simulink model "MODEL_TEMPLATE_NonLinear_Tire"  (Simulink 7.5)
settings: Solver=ode45  StartTime=0.0  StopTime=500  MaxStep=0.01  RelTol=1e-3
values from neighbouring files (symbols this model uses):
  U = NaN(2,nsteps)    [runscript.m]
undefined symbols (not defined in the file or in its folder): a, A, b, B, Caf, Car, Iz, m, steer_amplitude, tire_model_type
libraries: simulink x1
settings Model: Creator=snb10  LastModifiedBy=Matt
settings DataIOCC: SignalLoggingName=sigsOut
settings OptimizationCC: InlineInvariantSignals=on  InitFltsAndDblsToZero=on
settings DebuggingCC: SaveWithParameterizedLinksMsg=none  SignalResolutionControl=TryResolveAllWithWarning  SolverPrmCheckMsg=none  MultiTaskDSMMsg=warning  MultiTaskCondExecSysMsg=none  StrictBusMsg=None
settings HardwareCC: TargetUnknown=on
settings RTWCC: IncludeERTFirstTime=on
settings GRTTargetCC: TargetFcnLib=ansi_tfl_tmw.mat

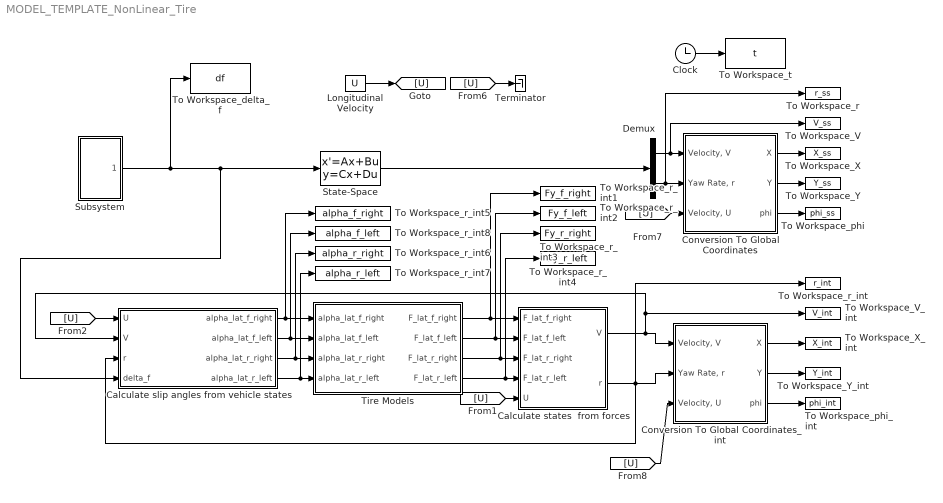
== system MODEL_TEMPLATE_NonLinear_Tire ==
  Calculate slip angles from vehicle states : Subsystem
  Calculate states  from forces : Subsystem
  Clock : Clock
      settings: Decimation=10
  Conversion To Global Coordinates : Subsystem
  Conversion To Global Coordinates_int : Subsystem
  Demux : Demux  Outputs=2
  Longitudinal Velocity : Constant  Value=U  OutDataType=sfix(16)  OutScaling=2^0
  State-Space : StateSpace  A=A  B=B(:,1)  C=eye(2)  D=zeros(2,1)
  Subsystem : Subsystem
  Terminator : Terminator
  Tire Models : Subsystem
  To Workspace_V : ToWorkspace  VariableName=V_ss  SampleTime=-1  SaveFormat=Array
  To Workspace_V_int : ToWorkspace  VariableName=V_int  SampleTime=-1  SaveFormat=Array
  To Workspace_X : ToWorkspace  VariableName=X_ss  SampleTime=-1  SaveFormat=Array
  To Workspace_X_int : ToWorkspace  VariableName=X_int  SampleTime=-1  SaveFormat=Array
  To Workspace_Y : ToWorkspace  VariableName=Y_ss  SampleTime=-1  SaveFormat=Array
  To Workspace_Y_int : ToWorkspace  VariableName=Y_int  SampleTime=-1  SaveFormat=Array
  To Workspace_delta_f : ToWorkspace  VariableName=df  SampleTime=-1  SaveFormat=Array
  To Workspace_phi : ToWorkspace  VariableName=phi_ss  SampleTime=-1  SaveFormat=Array
  To Workspace_phi_int : ToWorkspace  VariableName=phi_int  SampleTime=-1  SaveFormat=Array
  To Workspace_r : ToWorkspace  VariableName=r_ss  SampleTime=-1  SaveFormat=Array
  To Workspace_r_int : ToWorkspace  VariableName=r_int  SampleTime=-1  SaveFormat=Array
  To Workspace_r_int1 : ToWorkspace  VariableName=Fy_f_right  SampleTime=-1  SaveFormat=Array
  To Workspace_r_int2 : ToWorkspace  VariableName=Fy_f_left  SampleTime=-1  SaveFormat=Array
  To Workspace_r_int3 : ToWorkspace  VariableName=Fy_r_right  SampleTime=-1  SaveFormat=Array
  To Workspace_r_int4 : ToWorkspace  VariableName=Fy_r_left  SampleTime=-1  SaveFormat=Array
  To Workspace_r_int5 : ToWorkspace  VariableName=alpha_f_right  SampleTime=-1  SaveFormat=Array
  To Workspace_r_int6 : ToWorkspace  VariableName=alpha_r_right  SampleTime=-1  SaveFormat=Array
  To Workspace_r_int7 : ToWorkspace  VariableName=alpha_r_left  SampleTime=-1  SaveFormat=Array
  To Workspace_r_int8 : ToWorkspace  VariableName=alpha_f_left  SampleTime=-1  SaveFormat=Array
  To Workspace_t : ToWorkspace  VariableName=t  SampleTime=-1  SaveFormat=Array
  wires:
  Demux/1 -> Conversion To Global Coordinates/1("Velocity, V"), To Workspace_V/1
  Conversion To Global Coordinates/1(X) -> To Workspace_X/1
  Conversion To Global Coordinates/2(Y) -> To Workspace_Y/1
  Demux/2 -> Conversion To Global Coordinates/2("Yaw Rate, r"), To Workspace_r/1
  State-Space/1 -> Demux/1
  [U] -> Conversion To Global Coordinates/3("Velocity, U")
  Conversion To Global Coordinates/3(phi) -> To Workspace_phi/1
  Subsystem/1(delta_f) -> To Workspace_delta_f/1, State-Space/1, Calculate slip angles from vehicle states/4(delta_f)
  Clock/1 -> To Workspace_t/1
  Calculate states  from forces/1(V) -> Conversion To Global Coordinates_int/1("Velocity, V"), To Workspace_V_int/1, Calculate slip angles from vehicle states/2(V)
  Conversion To Global Coordinates_int/1(X) -> To Workspace_X_int/1
  Conversion To Global Coordinates_int/2(Y) -> To Workspace_Y_int/1
  [U] -> Conversion To Global Coordinates_int/3("Velocity, U")
  Conversion To Global Coordinates_int/3(phi) -> To Workspace_phi_int/1
  Longitudinal Velocity/1 -> [U]
  [U] -> Terminator/1
  Calculate states  from forces/2(r) -> To Workspace_r_int/1, Conversion To Global Coordinates_int/2("Yaw Rate, r"), Calculate slip angles from vehicle states/3(r)
  Tire Models/1(F_lat_f_right) -> Calculate states  from forces/1(F_lat_f_right), To Workspace_r_int1/1
  Calculate slip angles from vehicle states/1(alpha_lat_f_right) -> To Workspace_r_int5/1, Tire Models/1(alpha_lat_f_right)
  [U] -> Calculate states  from forces/5(U)
  Tire Models/2(F_lat_f_left) -> Calculate states  from forces/2(F_lat_f_left), To Workspace_r_int2/1
  Tire Models/3(F_lat_r_right) -> Calculate states  from forces/3(F_lat_r_right), To Workspace_r_int3/1
  Tire Models/4(F_lat_r_left) -> Calculate states  from forces/4(F_lat_r_left), To Workspace_r_int4/1
  Calculate slip angles from vehicle states/2(alpha_lat_f_left) -> To Workspace_r_int8/1, Tire Models/2(alpha_lat_f_left)
  Calculate slip angles from vehicle states/3(alpha_lat_r_right) -> To Workspace_r_int6/1, Tire Models/3(alpha_lat_r_right)
  Calculate slip angles from vehicle states/4(alpha_lat_r_left) -> To Workspace_r_int7/1, Tire Models/4(alpha_lat_r_left)
  [U] -> Calculate slip angles from vehicle states/1(U)

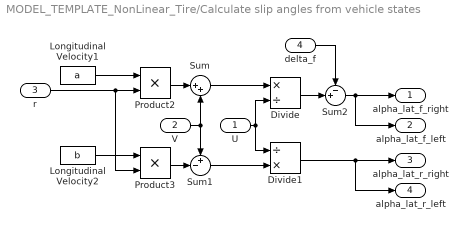
== system MODEL_TEMPLATE_NonLinear_Tire/Calculate slip angles from vehicle states ==
  U : Inport  OutDataType=sfix(16)  OutScaling=2^0
  V : Inport  Port=2  OutDataType=sfix(16)  OutScaling=2^0
  r : Inport  Port=3  OutDataType=sfix(16)  OutScaling=2^0
  delta_f : Inport  Port=4  OutDataType=sfix(16)  OutScaling=2^0
  Divide : Product  Inputs=*/  OutDataType=sfix(16)  OutScaling=2^-10
  Divide1 : Product  Inputs=/*  OutDataType=sfix(16)  OutScaling=2^-10
  Longitudinal Velocity1 : Constant  Value=a  OutDataType=sfix(16)  OutScaling=2^0
  Longitudinal Velocity2 : Constant  Value=b  OutDataType=sfix(16)  OutScaling=2^0
  Product2 : Product  OutDataType=sfix(16)  OutScaling=2^0  RndMeth=Zero
  Product3 : Product  OutDataType=sfix(16)  OutScaling=2^0  RndMeth=Zero
  Sum : Sum  Inputs=|++  OutDataType=sfix(16)  OutScaling=2^0
  Sum1 : Sum  Inputs=+-|  OutDataType=sfix(16)  OutScaling=2^0
  Sum2 : Sum  Inputs=-+|  OutDataType=sfix(16)  OutScaling=2^0
  alpha_lat_f_right : Outport  OutDataType=sfix(16)  OutScaling=2^0
  alpha_lat_f_left : Outport  Port=2  OutDataType=sfix(16)  OutScaling=2^0
  alpha_lat_r_right : Outport  Port=3  OutDataType=sfix(16)  OutScaling=2^0
  alpha_lat_r_left : Outport  Port=4  OutDataType=sfix(16)  OutScaling=2^0
  wires:
  Longitudinal Velocity2/1 -> Product3/1
  delta_f/1 -> Sum2/1
  r/1 -> Product2/2, Product3/2
  Longitudinal Velocity1/1 -> Product2/1
  Product2/1 -> Sum/1
  V/1 -> Sum/2, Sum1/1
  Product3/1 -> Sum1/2
  Sum/1 -> Divide/1
  U/1 -> Divide/2, Divide1/1
  Sum1/1 -> Divide1/2
  Divide/1 -> Sum2/2
  Sum2/1 -> alpha_lat_f_right/1, alpha_lat_f_left/1
  Divide1/1 -> alpha_lat_r_right/1, alpha_lat_r_left/1

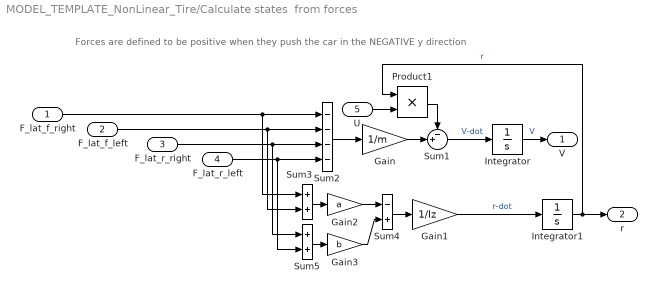
== system MODEL_TEMPLATE_NonLinear_Tire/Calculate states  from forces ==
  note: Forces are defined to be positive when they push the car in the NEGATIVE y direction
  F_lat_f_right : Inport  OutDataType=sfix(16)  OutScaling=2^0
  F_lat_f_left : Inport  Port=2  OutDataType=sfix(16)  OutScaling=2^0
  F_lat_r_right : Inport  Port=3  OutDataType=sfix(16)  OutScaling=2^0
  F_lat_r_left : Inport  Port=4  OutDataType=sfix(16)  OutScaling=2^0
  U : Inport  Port=5  OutDataType=sfix(16)  OutScaling=2^0
  Gain : Gain  Gain=1/m  ParameterDataType=sfix(16)  ParameterScaling=2^0  OutDataType=sfix(16)  OutScaling=2^0
  Gain1 : Gain  Gain=1/Iz  ParameterDataType=sfix(16)  ParameterScaling=2^0  OutDataType=sfix(16)  OutScaling=2^0
  Gain2 : Gain  Gain=a  ParameterDataType=sfix(16)  ParameterScaling=2^0  OutDataType=sfix(16)  OutScaling=2^0
  Gain3 : Gain  Gain=b  ParameterDataType=sfix(16)  ParameterScaling=2^0  OutDataType=sfix(16)  OutScaling=2^0
  Integrator : Integrator
  Integrator1 : Integrator
  Product1 : Product  OutDataType=sfix(16)  OutScaling=2^0  RndMeth=Zero
  Sum1 : Sum  Inputs=-+|  OutDataType=sfix(16)  OutScaling=2^0  SaturateOnIntegerOverflow=on
  Sum2 : Sum  Inputs=----  OutDataType=sfix(16)  OutScaling=2^0  SaturateOnIntegerOverflow=on
  Sum3 : Sum  OutDataType=sfix(16)  OutScaling=2^0  SaturateOnIntegerOverflow=on
  Sum4 : Sum  Inputs=-+  OutDataType=sfix(16)  OutScaling=2^0  SaturateOnIntegerOverflow=on
  Sum5 : Sum  OutDataType=sfix(16)  OutScaling=2^0  SaturateOnIntegerOverflow=on
  V : Outport  OutDataType=sfix(16)  OutScaling=2^0
  r : Outport  Port=2  OutDataType=sfix(16)  OutScaling=2^0
  wires:
  Gain/1 -> Sum1/2
  Sum1/1 -> Integrator/1  "V-dot"
  U/1 -> Product1/2
  Product1/1 -> Sum1/1
  Sum2/1 -> Gain/1
  Gain1/1 -> Integrator1/1  "r-dot"
  Sum4/1 -> Gain1/1
  Sum3/1 -> Gain2/1
  Gain2/1 -> Sum4/1
  Gain3/1 -> Sum4/2
  Sum5/1 -> Gain3/1
  Integrator/1 -> V/1  "V"
  F_lat_f_right/1 -> Sum2/1, Sum3/1
  F_lat_f_left/1 -> Sum2/2, Sum3/2
  F_lat_r_right/1 -> Sum2/3, Sum5/1
  F_lat_r_left/1 -> Sum2/4, Sum5/2
  Integrator1/1 -> Product1/1, r/1  "r"

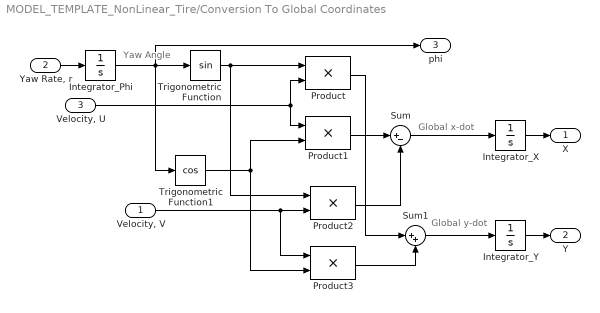
== system MODEL_TEMPLATE_NonLinear_Tire/Conversion To Global Coordinates ==
  note: Yaw Angle
  note: Global x-dot
  note: Global y-dot
  "Velocity, V" : Inport  OutDataType=sfix(16)  OutScaling=2^0
  "Yaw Rate, r" : Inport  Port=2  OutDataType=sfix(16)  OutScaling=2^0
  "Velocity, U" : Inport  Port=3  OutDataType=sfix(16)  OutScaling=2^0
  Integrator_Phi : Integrator
  Integrator_X : Integrator
  Integrator_Y : Integrator
  Product{,1..3} (4 alike) : Product  OutDataType=sfix(16)  OutScaling=2^0  SaturateOnIntegerOverflow=on  OutDataTypeStr=Inherit: Same as first input
  Sum : Sum  Inputs=|+-  OutDataType=sfix(16)  OutScaling=2^0  SaturateOnIntegerOverflow=on
  Sum1 : Sum  Inputs=|++  OutDataType=sfix(16)  OutScaling=2^0  SaturateOnIntegerOverflow=on
  Trigonometric Function : Trigonometry
  Trigonometric Function1 : Trigonometry  Operator=cos
  X : Outport  OutDataType=sfix(16)  OutScaling=2^0
  Y : Outport  Port=2  OutDataType=sfix(16)  OutScaling=2^0
  phi : Outport  Port=3  OutDataType=sfix(16)  OutScaling=2^0
  wires:
  Integrator_Phi/1 -> Trigonometric Function/1, Trigonometric Function1/1, phi/1
  "Velocity, U"/1 -> Product/2, Product1/1
  "Velocity, V"/1 -> Product2/2, Product3/1
  Trigonometric Function1/1 -> Product1/2, Product3/2
  Product1/1 -> Sum/1
  Product2/1 -> Sum/2
  Trigonometric Function/1 -> Product/1, Product2/1
  Sum/1 -> Integrator_X/1
  Product/1 -> Sum1/1
  Product3/1 -> Sum1/2
  Sum1/1 -> Integrator_Y/1
  "Yaw Rate, r"/1 -> Integrator_Phi/1
  Integrator_X/1 -> X/1
  Integrator_Y/1 -> Y/1

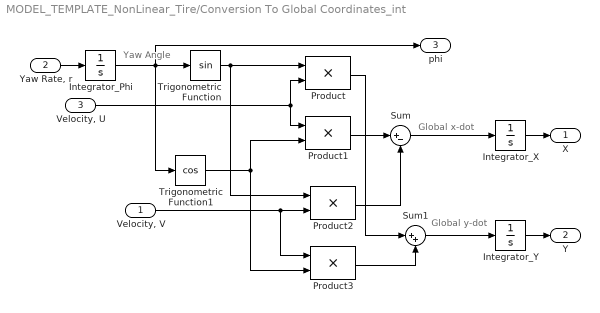
== system MODEL_TEMPLATE_NonLinear_Tire/Conversion To Global Coordinates_int ==
  note: Global y-dot
  note: Global x-dot
  note: Yaw Angle
  "Velocity, V" : Inport  OutDataType=sfix(16)  OutScaling=2^0
  "Yaw Rate, r" : Inport  Port=2  OutDataType=sfix(16)  OutScaling=2^0
  "Velocity, U" : Inport  Port=3  OutDataType=sfix(16)  OutScaling=2^0
  Integrator_Phi : Integrator
  Integrator_X : Integrator
  Integrator_Y : Integrator
  Product{,1..3} (4 alike) : Product  OutDataType=sfix(16)  OutScaling=2^0  SaturateOnIntegerOverflow=on  OutDataTypeStr=Inherit: Same as first input
  Sum : Sum  Inputs=|+-  OutDataType=sfix(16)  OutScaling=2^0  SaturateOnIntegerOverflow=on
  Sum1 : Sum  Inputs=|++  OutDataType=sfix(16)  OutScaling=2^0  SaturateOnIntegerOverflow=on
  Trigonometric Function : Trigonometry
  Trigonometric Function1 : Trigonometry  Operator=cos
  X : Outport  OutDataType=sfix(16)  OutScaling=2^0
  Y : Outport  Port=2  OutDataType=sfix(16)  OutScaling=2^0
  phi : Outport  Port=3  OutDataType=sfix(16)  OutScaling=2^0
  wires:
  Integrator_Y/1 -> Y/1
  Integrator_X/1 -> X/1
  "Yaw Rate, r"/1 -> Integrator_Phi/1
  Sum1/1 -> Integrator_Y/1
  Product3/1 -> Sum1/2
  Product/1 -> Sum1/1
  Sum/1 -> Integrator_X/1
  Trigonometric Function/1 -> Product2/1, Product/1
  Product2/1 -> Sum/2
  Product1/1 -> Sum/1
  Trigonometric Function1/1 -> Product3/2, Product1/2
  "Velocity, V"/1 -> Product3/1, Product2/2
  "Velocity, U"/1 -> Product1/1, Product/2
  Integrator_Phi/1 -> phi/1, Trigonometric Function1/1, Trigonometric Function/1

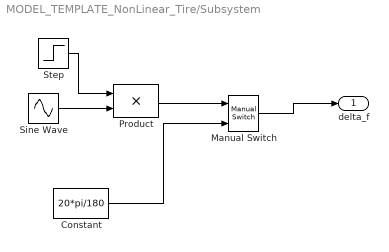
== system MODEL_TEMPLATE_NonLinear_Tire/Subsystem ==
  Constant : Constant  Value=20*pi/180  OutDataType=sfix(16)  OutScaling=2^0
  Manual Switch : simulink/Signal Routing/Manual Switch  SystemSampleTime=-1  sw=1  action=0  varsize=off
  Product : Product  OutDataType=sfix(16)  OutScaling=2^0  SaturateOnIntegerOverflow=on  OutDataTypeStr=Inherit: Same as first input
  Sine Wave : Sin  Amplitude=steer_amplitude  Bias=0  Frequency=0.1*2*pi  Phase=0  Samples=10  SampleTime=0  Offset=0
  Step : Step  Time=10  Before=1  After=0  SampleTime=0
  delta_f : Outport  OutDataType=sfix(16)  OutScaling=2^0
  wires:
  Step/1 -> Product/1
  Sine Wave/1 -> Product/2
  Constant/1 -> Manual Switch/2
  Product/1 -> Manual Switch/1
  Manual Switch/1 -> delta_f/1

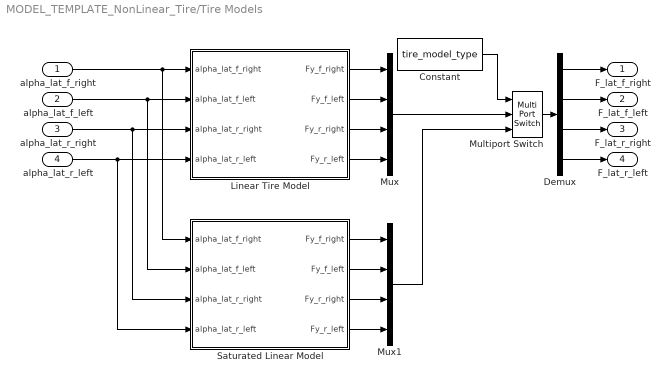
== system MODEL_TEMPLATE_NonLinear_Tire/Tire Models ==
  alpha_lat_f_right : Inport
  alpha_lat_f_left : Inport  Port=2
  alpha_lat_r_right : Inport  Port=3
  alpha_lat_r_left : Inport  Port=4
  Constant : Constant  Value=tire_model_type  OutDataType=fixdt(1, 16)  OutScaling=2^0
  Demux : Demux
  Linear Tire Model : Subsystem
  Multiport Switch : MultiPortSwitch  Inputs=2  zeroidx=off  OutDataType=fixdt(1, 16)  OutScaling=2^0
  Mux : Mux
  Mux1 : Mux
  Saturated Linear Model : Subsystem
  F_lat_f_right : Outport
  F_lat_f_left : Outport  Port=2
  F_lat_r_right : Outport  Port=3
  F_lat_r_left : Outport  Port=4
  wires:
  alpha_lat_f_right/1 -> Linear Tire Model/1(alpha_lat_f_right), Saturated Linear Model/1(alpha_lat_f_right)
  alpha_lat_f_left/1 -> Linear Tire Model/2(alpha_lat_f_left), Saturated Linear Model/2(alpha_lat_f_left)
  alpha_lat_r_right/1 -> Linear Tire Model/3(alpha_lat_r_right), Saturated Linear Model/3(alpha_lat_r_right)
  alpha_lat_r_left/1 -> Linear Tire Model/4(alpha_lat_r_left), Saturated Linear Model/4(alpha_lat_r_left)
  Linear Tire Model/1(Fy_f_right) -> Mux/1
  Linear Tire Model/2(Fy_f_left) -> Mux/2
  Linear Tire Model/3(Fy_r_right) -> Mux/3
  Linear Tire Model/4(Fy_r_left) -> Mux/4
  Saturated Linear Model/1(Fy_f_right) -> Mux1/1
  Saturated Linear Model/2(Fy_f_left) -> Mux1/2
  Saturated Linear Model/3(Fy_r_right) -> Mux1/3
  Saturated Linear Model/4(Fy_r_left) -> Mux1/4
  Demux/1 -> F_lat_f_right/1
  Demux/2 -> F_lat_f_left/1
  Demux/3 -> F_lat_r_right/1
  Demux/4 -> F_lat_r_left/1
  Mux/1 -> Multiport Switch/2
  Mux1/1 -> Multiport Switch/3
  Constant/1 -> Multiport Switch/1
  Multiport Switch/1 -> Demux/1

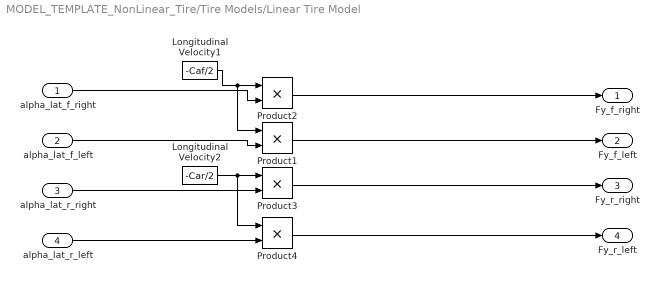
== system MODEL_TEMPLATE_NonLinear_Tire/Tire Models/Linear Tire Model ==
  alpha_lat_f_right : Inport  OutDataType=sfix(16)  OutScaling=2^0
  alpha_lat_f_left : Inport  Port=2  OutDataType=sfix(16)  OutScaling=2^0
  alpha_lat_r_right : Inport  Port=3  OutDataType=sfix(16)  OutScaling=2^0
  alpha_lat_r_left : Inport  Port=4  OutDataType=sfix(16)  OutScaling=2^0
  Longitudinal Velocity1 : Constant  Value=-Caf/2  OutDataType=sfix(16)  OutScaling=2^0
  Longitudinal Velocity2 : Constant  Value=-Car/2  OutDataType=sfix(16)  OutScaling=2^0
  Product{1..4} (4 alike) : Product  OutDataType=sfix(16)  OutScaling=2^0  RndMeth=Zero
  Fy_f_right : Outport  OutDataType=sfix(16)  OutScaling=2^0
  Fy_f_left : Outport  Port=2  OutDataType=sfix(16)  OutScaling=2^0
  Fy_r_right : Outport  Port=3  OutDataType=sfix(16)  OutScaling=2^0
  Fy_r_left : Outport  Port=4  OutDataType=sfix(16)  OutScaling=2^0
  wires:
  alpha_lat_f_right/1 -> Product2/2
  alpha_lat_f_left/1 -> Product1/2
  alpha_lat_r_right/1 -> Product3/2
  alpha_lat_r_left/1 -> Product4/2
  Longitudinal Velocity1/1 -> Product1/1, Product2/1
  Longitudinal Velocity2/1 -> Product4/1, Product3/1
  Product2/1 -> Fy_f_right/1
  Product1/1 -> Fy_f_left/1
  Product3/1 -> Fy_r_right/1
  Product4/1 -> Fy_r_left/1

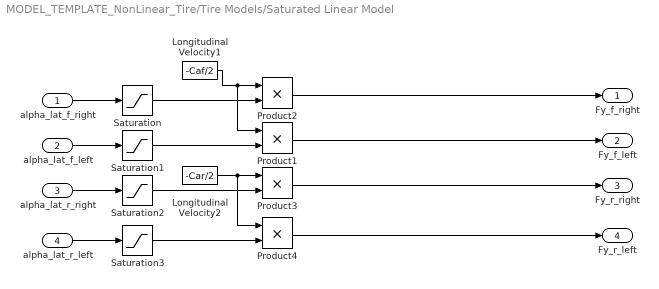
== system MODEL_TEMPLATE_NonLinear_Tire/Tire Models/Saturated Linear Model ==
  alpha_lat_f_right : Inport  OutDataType=sfix(16)  OutScaling=2^0
  alpha_lat_f_left : Inport  Port=2  OutDataType=sfix(16)  OutScaling=2^0
  alpha_lat_r_right : Inport  Port=3  OutDataType=sfix(16)  OutScaling=2^0
  alpha_lat_r_left : Inport  Port=4  OutDataType=sfix(16)  OutScaling=2^0
  Longitudinal Velocity1 : Constant  Value=-Caf/2  OutDataType=sfix(16)  OutScaling=2^0
  Longitudinal Velocity2 : Constant  Value=-Car/2  OutDataType=sfix(16)  OutScaling=2^0
  Product{1..4} (4 alike) : Product  OutDataType=sfix(16)  OutScaling=2^0  RndMeth=Zero
  Saturation{,1..3} (4 alike) : Saturate  UpperLimit=5*pi/180  LowerLimit=-5*pi/180  OutDataType=fixdt(1, 16)  OutScaling=2^0
  Fy_f_right : Outport  OutDataType=sfix(16)  OutScaling=2^0
  Fy_f_left : Outport  Port=2  OutDataType=sfix(16)  OutScaling=2^0
  Fy_r_right : Outport  Port=3  OutDataType=sfix(16)  OutScaling=2^0
  Fy_r_left : Outport  Port=4  OutDataType=sfix(16)  OutScaling=2^0
  wires:
  Product4/1 -> Fy_r_left/1
  Product3/1 -> Fy_r_right/1
  Product1/1 -> Fy_f_left/1
  Product2/1 -> Fy_f_right/1
  Longitudinal Velocity2/1 -> Product3/1, Product4/1
  Longitudinal Velocity1/1 -> Product2/1, Product1/1
  alpha_lat_f_right/1 -> Saturation/1
  Saturation/1 -> Product2/2
  alpha_lat_f_left/1 -> Saturation1/1
  alpha_lat_r_right/1 -> Saturation2/1
  alpha_lat_r_left/1 -> Saturation3/1
  Saturation1/1 -> Product1/2
  Saturation2/1 -> Product3/2
  Saturation3/1 -> Product4/2
